simulink model "slidingSimulSaturado"  (R2017a)
settings: Solver=VariableStepAuto  StartTime=0.0  StopTime=tSimul  RelTol=1e-3
values from neighbouring files (symbols this model uses):
  Acont = [0 1;0 0]    [slidingPL.m]    (also in slidingSaturado.m)
  aLB = -1.5    [slidingPL.m]    (also in slidingSaturado.m)
  aUB = 1.0    (= 1)    [slidingPL.m]    (also in slidingSaturado.m)
  Bcont = [0;1]    [slidingPL.m]    (also in slidingSaturado.m)
  Ccont = eye(2)    [slidingPL.m]    (also in slidingSaturado.m)
  d = 0    [slidingPL.m]    (also in slidingSaturado.m)
  Dcont = [0;0]    [slidingPL.m]    (also in slidingSaturado.m)
  Ldes = 2    [slidingPL.m]    (also in slidingSaturado.m)
  meanError = -0.0091    [slidingPL.m]    (also in slidingSaturado.m)
  perf = input('Tipo de lider (perfecto(1), ruidoso(0)):')    [slidingPL.m]    (also in slidingSaturado.m)
  ts = 0.1    [slidingPL.m]    (also in slidingSaturado.m)
  v0Bici1 = 1    [slidingPL.m]    (also in slidingSaturado.m)
  v0Bici2 = 1    [slidingPL.m]    (also in slidingSaturado.m)
  v0Bici3 = 1    [slidingPL.m]    (also in slidingSaturado.m)
  v0Leader = input('Velocidad lider (m/s)(2.7,4.16,5)')    [slidingPL.m]    (also in slidingSaturado.m)
  varError = varError^2    (= 0.15800625)    [slidingPL.m]    (also in slidingSaturado.m)
  x0Bici1 = -10    [slidingPL.m]    (also in slidingSaturado.m)
  x0Bici2 = -20    [slidingPL.m]    (also in slidingSaturado.m)
  x0Bici3 = -30    [slidingPL.m]    (also in slidingSaturado.m)
  x0Leader = 0    [slidingPL.m]    (also in slidingSaturado.m)
undefined symbols (not defined in the file or in its folder): slidingFunction
settings Model: Creator=tlara  LastModifiedBy=tlara

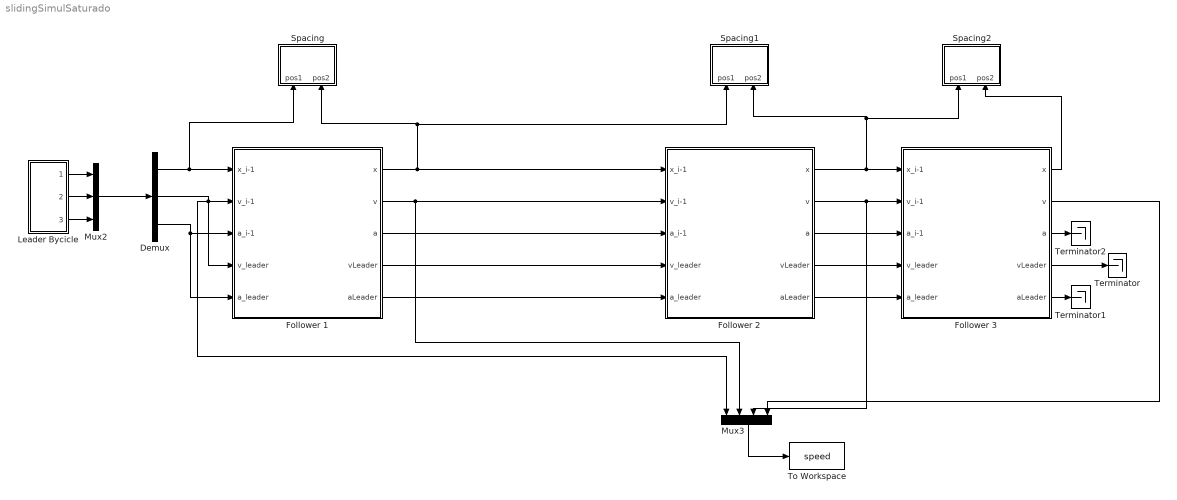
== system slidingSimulSaturado ==
  Demux : Demux  Outputs=3
  "Follower 1 " : Subsystem
  Follower 2 : Subsystem
  "Follower 3 " : Subsystem
  "Leader Bycicle " : Subsystem
  Mux2 : Mux  Inputs=3
  Mux3 : Mux
  Spacing : Subsystem
  Spacing1 : Subsystem
  Spacing2 : Subsystem
  Terminator : Terminator
  Terminator1 : Terminator
  Terminator2 : Terminator
  To Workspace : ToWorkspace  VariableName=speed  SaveFormat=Timeseries  SampleTime=-1
  wires:
  Demux/3 -> "Follower 1 "/5(a_leader), "Follower 1 "/3(a_i-1)
  Demux/2 -> Mux3/1, "Follower 1 "/4(v_leader), "Follower 1 "/2(v_i-1)
  Demux/1 -> Spacing/1(pos1), "Follower 1 "/1("x_i-1 ")
  "Follower 1 "/1(x) -> Spacing1/1(pos1), Spacing/2(pos2), Follower 2/1("x_i-1 ")
  "Follower 1 "/2(v) -> Follower 2/2(v_i-1), Mux3/2
  "Follower 1 "/3(a) -> Follower 2/3(a_i-1)
  "Follower 1 "/4("vLeader ") -> Follower 2/4(v_leader)
  "Follower 1 "/5(aLeader) -> Follower 2/5(a_leader)
  Follower 2/1(x) -> Spacing2/1(pos1), Spacing1/2(pos2), "Follower 3 "/1("x_i-1 ")
  Follower 2/2(v) -> Mux3/3, "Follower 3 "/2(v_i-1)
  Follower 2/3(a) -> "Follower 3 "/3(a_i-1)
  Follower 2/4("vLeader ") -> "Follower 3 "/4(v_leader)
  Follower 2/5(aLeader) -> "Follower 3 "/5(a_leader)
  "Leader Bycicle "/1(Position) -> Mux2/1
  "Leader Bycicle "/2(Speed) -> Mux2/2
  "Leader Bycicle "/3("Acceleration ") -> Mux2/3
  Mux2/1 -> Demux/1
  "Follower 3 "/1(x) -> Spacing2/2(pos2)
  "Follower 3 "/4("vLeader ") -> Terminator/1
  "Follower 3 "/5(aLeader) -> Terminator1/1
  "Follower 3 "/3(a) -> Terminator2/1
  Mux3/1 -> To Workspace/1
  "Follower 3 "/2(v) -> Mux3/4

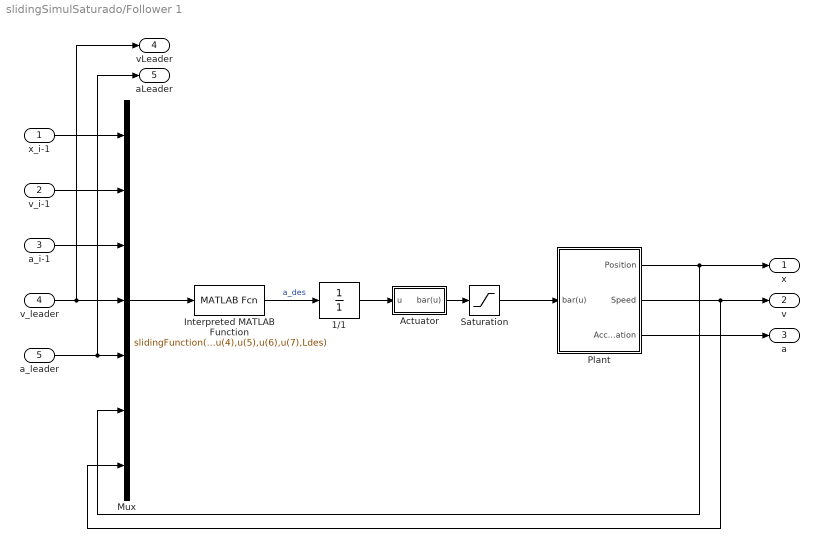
== system slidingSimulSaturado/Follower 1  ==
  "x_i-1 " : Inport
  v_i-1 : Inport  Port=2
  a_i-1 : Inport  Port=3
  v_leader : Inport  Port=4
  a_leader : Inport  Port=5
  "1/1 " : DiscreteTransferFcn  Denominator=[1]  SampleTime=ts
  Actuator : Subsystem
  Interpreted MATLAB Function : MATLABFcn  MATLABFcn=slidingFunction(u(1),u(2),u(3),u(4),u(5),u(6),u(7),Ldes)  OutputDimensions=1
  Mux : Mux  Inputs=7
  Plant : Subsystem
  Saturation : Saturate  UpperLimit=aUB  LowerLimit=aLB
  x : Outport
  v : Outport  Port=2
  a : Outport  Port=3
  "vLeader " : Outport  Port=4
  aLeader : Outport  Port=5
  wires:
  Interpreted MATLAB Function/1 -> "1/1 "/1  "a_des"
  Mux/1 -> Interpreted MATLAB Function/1
  "x_i-1 "/1 -> Mux/1
  v_i-1/1 -> Mux/2
  a_i-1/1 -> Mux/3
  v_leader/1 -> "vLeader "/1, Mux/4
  a_leader/1 -> aLeader/1, Mux/5
  Actuator/1(bar(u)) -> Saturation/1
  Saturation/1 -> Plant/1(bar(u))
  Plant/3(Acceleration) -> a/1
  Plant/2("Speed ") -> Mux/7, v/1
  Plant/1(Position) -> Mux/6, x/1
  "1/1 "/1 -> Actuator/1(u)

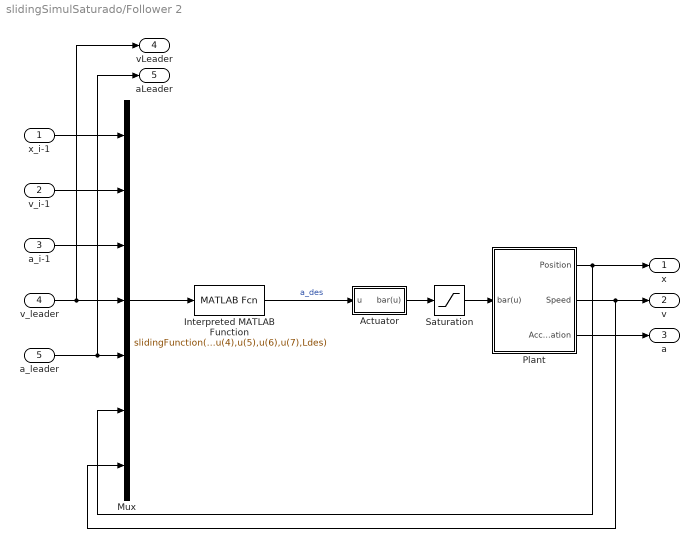
== system slidingSimulSaturado/Follower 2 ==
  "x_i-1 " : Inport
  v_i-1 : Inport  Port=2
  a_i-1 : Inport  Port=3
  v_leader : Inport  Port=4
  a_leader : Inport  Port=5
  Actuator : Subsystem
  Interpreted MATLAB Function : MATLABFcn  MATLABFcn=slidingFunction(u(1),u(2),u(3),u(4),u(5),u(6),u(7),Ldes)  OutputDimensions=1
  Mux : Mux  Inputs=7
  Plant : Subsystem
  Saturation : Saturate  UpperLimit=aUB  LowerLimit=aLB
  x : Outport
  v : Outport  Port=2
  a : Outport  Port=3
  "vLeader " : Outport  Port=4
  aLeader : Outport  Port=5
  wires:
  Interpreted MATLAB Function/1 -> Actuator/1(u)  "a_des"
  Plant/1(Position) -> Mux/6, x/1
  Mux/1 -> Interpreted MATLAB Function/1
  "x_i-1 "/1 -> Mux/1
  v_i-1/1 -> Mux/2
  a_i-1/1 -> Mux/3
  v_leader/1 -> "vLeader "/1, Mux/4
  a_leader/1 -> aLeader/1, Mux/5
  Actuator/1(bar(u)) -> Saturation/1
  Saturation/1 -> Plant/1(bar(u))
  Plant/2("Speed ") -> Mux/7, v/1
  Plant/3(Acceleration) -> a/1

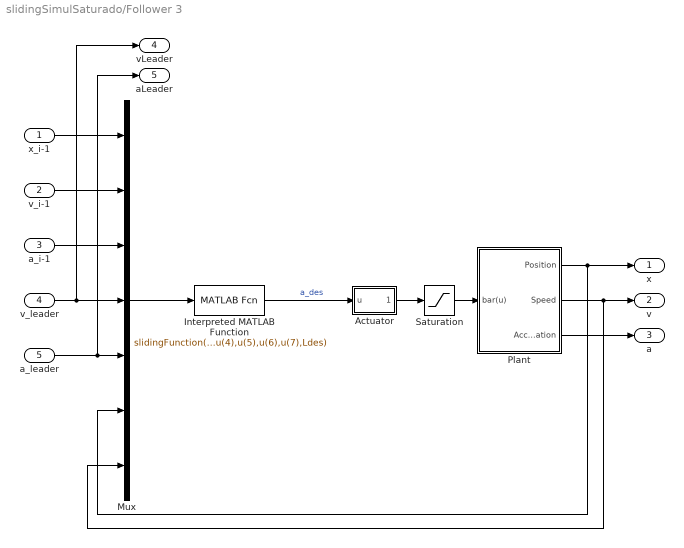
== system slidingSimulSaturado/Follower 3  ==
  "x_i-1 " : Inport
  v_i-1 : Inport  Port=2
  a_i-1 : Inport  Port=3
  v_leader : Inport  Port=4
  a_leader : Inport  Port=5
  Actuator : Subsystem
  Interpreted MATLAB Function : MATLABFcn  MATLABFcn=slidingFunction(u(1),u(2),u(3),u(4),u(5),u(6),u(7),Ldes)  OutputDimensions=1
  Mux : Mux  Inputs=7
  Plant : Subsystem
  Saturation : Saturate  UpperLimit=aUB  LowerLimit=aLB
  x : Outport
  v : Outport  Port=2
  a : Outport  Port=3
  "vLeader " : Outport  Port=4
  aLeader : Outport  Port=5
  wires:
  Interpreted MATLAB Function/1 -> Actuator/1(u)  "a_des"
  Mux/1 -> Interpreted MATLAB Function/1
  "x_i-1 "/1 -> Mux/1
  v_i-1/1 -> Mux/2
  a_i-1/1 -> Mux/3
  v_leader/1 -> "vLeader "/1, Mux/4
  a_leader/1 -> aLeader/1, Mux/5
  Saturation/1 -> Plant/1(bar(u))
  Actuator/1(bar(u)) -> Saturation/1
  Plant/1(Position) -> Mux/6, x/1
  Plant/2("Speed ") -> Mux/7, v/1
  Plant/3(Acceleration) -> a/1

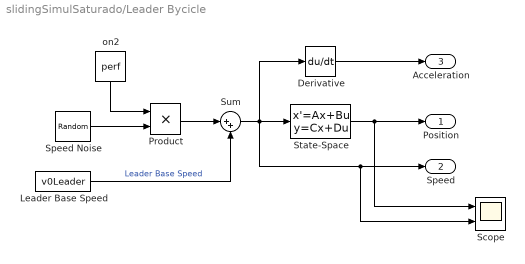
== system slidingSimulSaturado/Leader Bycicle  ==
  Derivative : Derivative
  "Leader Base Speed " : Constant  Value=v0Leader
  Product : Product
  Scope : Scope  NumInputPorts=2
  Speed Noise : RandomNumber  Variance=0.02  SampleTime=ts
  State-Space : StateSpace  A=[0]  B=[1]  C=[1]  D=[0]  X0=[x0Leader]  ContinuousStateAttributes='position'
  Sum : Sum  Inputs=|++
  on2 : Constant  Value=perf
  Position : Outport
  Speed : Outport  Port=2
  "Acceleration " : Outport  Port=3
  wires:
  "Leader Base Speed "/1 -> Sum/2  "Leader Base Speed"
  State-Space/1 -> Position/1, Scope/1
  Sum/1 -> Derivative/1, State-Space/1, Speed/1, Scope/2
  Derivative/1 -> "Acceleration "/1
  Product/1 -> Sum/1
  Speed Noise/1 -> Product/2
  on2/1 -> Product/1

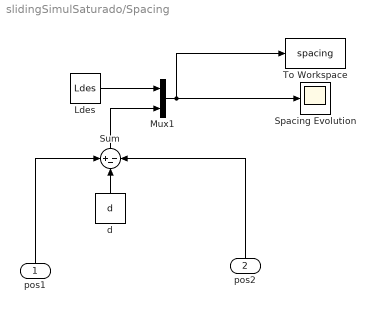
== system slidingSimulSaturado/Spacing ==
  pos1 : Inport
  pos2 : Inport  Port=2
  Ldes : Constant  Value=Ldes
  Mux1 : Mux  Inputs=2
  Spacing Evolution : Scope
  Sum : Sum  Inputs=+--
  To Workspace : ToWorkspace  VariableName=spacing  SaveFormat=Timeseries  SampleTime=-1
  "d " : Constant  Value=d
  wires:
  Ldes/1 -> Mux1/1
  "d "/1 -> Sum/2
  pos2/1 -> Sum/3
  pos1/1 -> Sum/1
  Sum/1 -> Mux1/2
  Mux1/1 -> To Workspace/1, Spacing Evolution/1

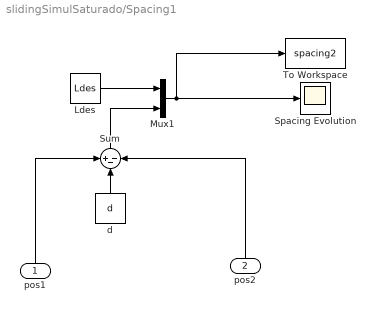
== system slidingSimulSaturado/Spacing1 ==
  pos1 : Inport
  pos2 : Inport  Port=2
  Ldes : Constant  Value=Ldes
  Mux1 : Mux  Inputs=2
  Spacing Evolution : Scope
  Sum : Sum  Inputs=+--
  To Workspace : ToWorkspace  VariableName=spacing2  SaveFormat=Timeseries  SampleTime=-1
  "d " : Constant  Value=d
  wires:
  Ldes/1 -> Mux1/1
  "d "/1 -> Sum/2
  pos2/1 -> Sum/3
  pos1/1 -> Sum/1
  Sum/1 -> Mux1/2
  Mux1/1 -> To Workspace/1, Spacing Evolution/1

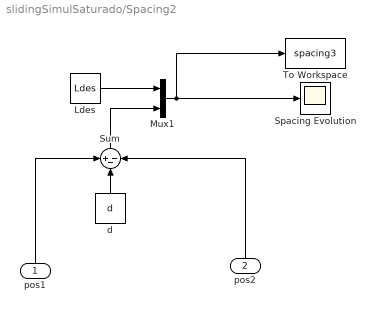
== system slidingSimulSaturado/Spacing2 ==
  pos1 : Inport
  pos2 : Inport  Port=2
  Ldes : Constant  Value=Ldes
  Mux1 : Mux  Inputs=2
  Spacing Evolution : Scope
  Sum : Sum  Inputs=+--
  To Workspace : ToWorkspace  VariableName=spacing3  SaveFormat=Timeseries  SampleTime=-1
  "d " : Constant  Value=d
  wires:
  Ldes/1 -> Mux1/1
  "d "/1 -> Sum/2
  pos2/1 -> Sum/3
  pos1/1 -> Sum/1
  Sum/1 -> Mux1/2
  Mux1/1 -> To Workspace/1, Spacing Evolution/1

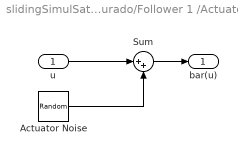
== system slidingSimulSaturado/Follower 1 /Actuator ==
  u : Inport
  Actuator Noise : RandomNumber  Mean=meanError  Variance=varError  SampleTime=ts
  Sum : Sum  Inputs=|++
  bar(u) : Outport
  wires:
  Sum/1 -> bar(u)/1
  u/1 -> Sum/1
  Actuator Noise/1 -> Sum/2

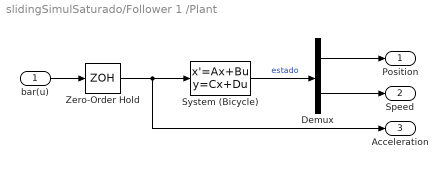
== system slidingSimulSaturado/Follower 1 /Plant ==
  bar(u) : Inport
  Demux : Demux  Outputs=2
  "System (Bicycle) " : StateSpace  A=Acont  B=Bcont  C=Ccont  D=Dcont  X0=[x0Bici1,v0Bici1]  ContinuousStateAttributes='Position'
  Zero-Order Hold : ZeroOrderHold  SampleTime=ts
  Position : Outport
  "Speed " : Outport  Port=2
  Acceleration : Outport  Port=3
  wires:
  bar(u)/1 -> Zero-Order Hold/1
  Zero-Order Hold/1 -> Acceleration/1, "System (Bicycle) "/1
  Demux/1 -> Position/1
  "System (Bicycle) "/1 -> Demux/1  "estado"
  Demux/2 -> "Speed "/1

== system slidingSimulSaturado/Follower 2/Actuator ==
  u : Inport
  Actuator Noise : RandomNumber  Mean=meanError  Variance=varError  SampleTime=ts
  Sum : Sum  Inputs=|++
  bar(u) : Outport
  wires:
  Sum/1 -> bar(u)/1
  u/1 -> Sum/1
  Actuator Noise/1 -> Sum/2

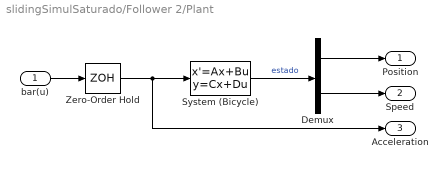
== system slidingSimulSaturado/Follower 2/Plant ==
  bar(u) : Inport
  Demux : Demux  Outputs=2
  "System (Bicycle) " : StateSpace  A=Acont  B=Bcont  C=Ccont  D=Dcont  X0=[x0Bici2,v0Bici2]  ContinuousStateAttributes='Position'
  Zero-Order Hold : ZeroOrderHold  SampleTime=ts
  Position : Outport
  "Speed " : Outport  Port=2
  Acceleration : Outport  Port=3
  wires:
  bar(u)/1 -> Zero-Order Hold/1
  Zero-Order Hold/1 -> Acceleration/1, "System (Bicycle) "/1
  Demux/1 -> Position/1
  "System (Bicycle) "/1 -> Demux/1  "estado"
  Demux/2 -> "Speed "/1

== system slidingSimulSaturado/Follower 3 /Actuator ==
  u : Inport
  Actuator Noise : RandomNumber  Mean=meanError  Variance=varError  SampleTime=ts
  Sum : Sum  Inputs=|++
  bar(u) : Outport
  wires:
  Sum/1 -> bar(u)/1
  u/1 -> Sum/1
  Actuator Noise/1 -> Sum/2

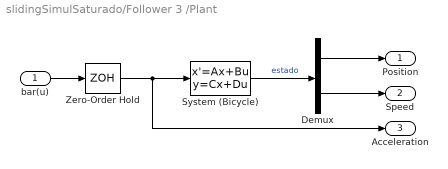
== system slidingSimulSaturado/Follower 3 /Plant ==
  bar(u) : Inport
  Demux : Demux  Outputs=2
  "System (Bicycle) " : StateSpace  A=Acont  B=Bcont  C=Ccont  D=Dcont  X0=[x0Bici3,v0Bici3]  ContinuousStateAttributes='Position'
  Zero-Order Hold : ZeroOrderHold  SampleTime=ts
  Position : Outport
  "Speed " : Outport  Port=2
  Acceleration : Outport  Port=3
  wires:
  bar(u)/1 -> Zero-Order Hold/1
  Zero-Order Hold/1 -> Acceleration/1, "System (Bicycle) "/1
  Demux/1 -> Position/1
  "System (Bicycle) "/1 -> Demux/1  "estado"
  Demux/2 -> "Speed "/1
